simulink model "bary_source_seeking"  (R2017a)
settings: Solver=ode4  StartTime=0  StopTime=tf  FixedStep=1e-5  RelTol=1e-3
values from neighbouring files (symbols this model uses):
  lambda = t/T    [gentrajmodel_2Drobot.m]    (also in main.m = 1; sim_model.m = 1; source_estimation.m = sestimation_info.lambda)
  nu = 10    [main.m]    (also in sim_model.m; source_estimation.m = sestimation_info.nu)
  SAT_CONTROL = 10    [main.m]    (also in sim_model.m)
  T_cur = 1    [main.m]    (also in run_control_law.m = sestimation_info.T_cur; sim_model.m)
  T_traj = 1    [main.m]    (also in run_control_law.m = trajectory_info.T_traj; sim_model.m)
  traj_type = 1    [main.m]    (also in sim_model.m)
  x0 = [2; 2; 0; 1; 1; 1]    [main.m]    (also in sim_model.m)
undefined symbols (not defined in the file or in its folder): devval, is_sat, v_max, v_min, w_max
settings Model: Creator=brunolnetto  LastModifiedBy=brunolnetto

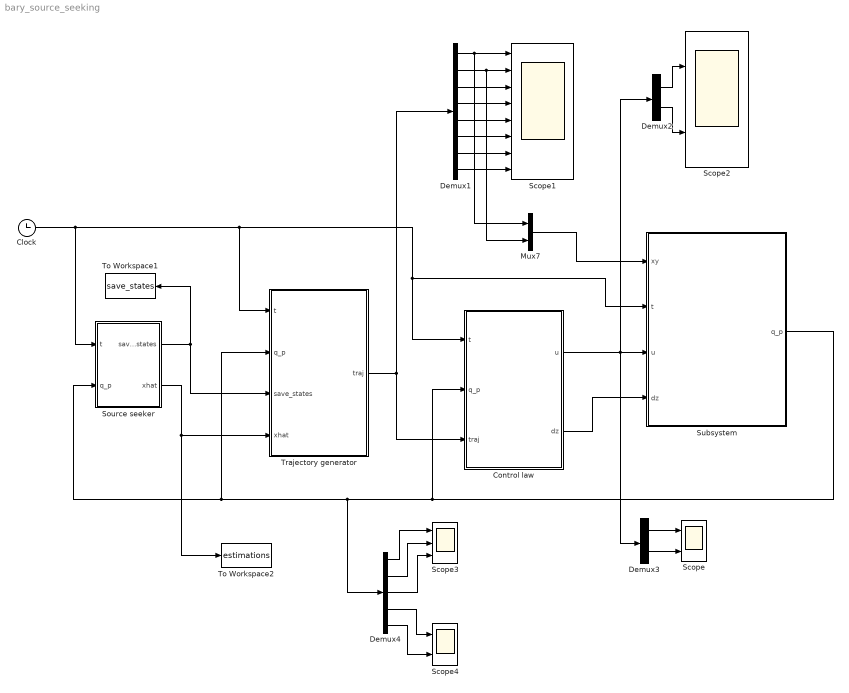
== system bary_source_seeking ==
  Clock : Clock
  Control law : MATLAB Function  TreatAsAtomicUnit=on
  Demux1 : Demux  Outputs=8
  Demux2 : Demux  Outputs=2
  Demux3 : Demux  Outputs=2
  Demux4 : Demux  Outputs=5
  Mux7 : Mux  Inputs=2
  Scope : Scope  NumInputPorts=2
  Scope1 : Scope  NumInputPorts=8
  Scope2 : Scope  NumInputPorts=2
  Scope3 : Scope  NumInputPorts=3
  Scope4 : Scope  NumInputPorts=2
  Source seeker : Subsystem
  Subsystem : Subsystem
  To Workspace1 : ToWorkspace  VariableName=save_states  SaveFormat=Structure With Time  SampleTime=-1
  To Workspace2 : ToWorkspace  VariableName=estimations  SaveFormat=Structure With Time  SampleTime=-1
  Trajectory generator : Subsystem
  wires:
  Clock/1 -> Control law/1(t), Subsystem/2(t), Trajectory generator/1(t), Source seeker/1(t)
  Demux1/3 -> Scope1/3
  Demux1/4 -> Scope1/4
  Demux1/5 -> Scope1/5
  Demux1/6 -> Scope1/6
  Demux1/7 -> Scope1/7
  Demux1/8 -> Scope1/8
  Demux1/2 -> Scope1/2, Mux7/2
  Demux1/1 -> Scope1/1, Mux7/1
  Mux7/1 -> Subsystem/1(xy)
  Control law/2(dz) -> Subsystem/4(dz)
  Source seeker/1(save_states) -> To Workspace1/1, Trajectory generator/3(save_states)
  Source seeker/2(xhat) -> Trajectory generator/4(xhat), To Workspace2/1
  Control law/1(u) -> Demux3/1, Demux2/1, Subsystem/3(u)
  Demux2/1 -> Scope2/1
  Demux2/2 -> Scope2/2
  Trajectory generator/1(traj) -> Demux1/1, Control law/3(traj)
  Demux3/1 -> Scope/1
  Demux3/2 -> Scope/2
  Subsystem/1(q_p) -> Control law/2(q_p), Demux4/1, Trajectory generator/2(q_p), Source seeker/2(q_p)
  Demux4/1 -> Scope3/1
  Demux4/2 -> Scope3/2
  Demux4/3 -> Scope3/3
  Demux4/4 -> Scope4/1
  Demux4/5 -> Scope4/2

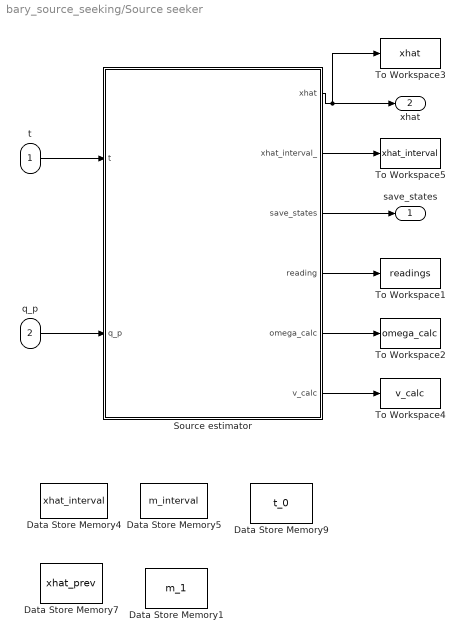
== system bary_source_seeking/Source seeker ==
  t : Inport
  q_p : Inport  Port=2
  Data Store Memory1 : DataStoreMemory  DataStoreName=m_1  ReadBeforeWriteMsg=warning  WriteAfterWriteMsg=warning  WriteAfterReadMsg=warning  ShowAdditionalParam=off  OutDataTypeStr=double
  Data Store Memory4 : DataStoreMemory  DataStoreName=xhat_interval  ReadBeforeWriteMsg=warning  WriteAfterWriteMsg=warning  WriteAfterReadMsg=warning  InitialValue=xhat0  ShowAdditionalParam=off  OutDataTypeStr=double  Dimensions=[2, 1]
  Data Store Memory5 : DataStoreMemory  DataStoreName=m_interval  ReadBeforeWriteMsg=warning  WriteAfterWriteMsg=warning  WriteAfterReadMsg=warning  ShowAdditionalParam=off  OutDataTypeStr=double
  Data Store Memory7 : DataStoreMemory  DataStoreName=xhat_prev  ReadBeforeWriteMsg=warning  WriteAfterWriteMsg=warning  WriteAfterReadMsg=warning  InitialValue=xhat0  ShowAdditionalParam=off  OutDataTypeStr=double
  Data Store Memory9 : DataStoreMemory  DataStoreName=t_0  ReadBeforeWriteMsg=warning  WriteAfterWriteMsg=warning  WriteAfterReadMsg=warning  ShowAdditionalParam=off  OutDataTypeStr=double
  Source estimator : MATLAB Function  TreatAsAtomicUnit=on
  To Workspace1 : ToWorkspace  VariableName=readings  SaveFormat=Structure With Time  SampleTime=-1
  To Workspace2 : ToWorkspace  VariableName=omega_calc  SaveFormat=Structure With Time  SampleTime=-1
  To Workspace3 : ToWorkspace  VariableName=xhat  SaveFormat=Structure With Time  SampleTime=-1
  To Workspace4 : ToWorkspace  VariableName=v_calc  SaveFormat=Structure With Time  SampleTime=-1
  To Workspace5 : ToWorkspace  VariableName=xhat_interval  SaveFormat=Structure With Time  SampleTime=-1
  save_states : Outport
  xhat : Outport  Port=2
  wires:
  Source estimator/4(reading) -> To Workspace1/1
  Source estimator/5(omega_calc) -> To Workspace2/1
  Source estimator/1(xhat) -> xhat/1, To Workspace3/1
  Source estimator/6(v_calc) -> To Workspace4/1
  t/1 -> Source estimator/1(t)
  q_p/1 -> Source estimator/2(q_p)
  Source estimator/3(save_states) -> save_states/1
  Source estimator/2(xhat_interval_) -> To Workspace5/1

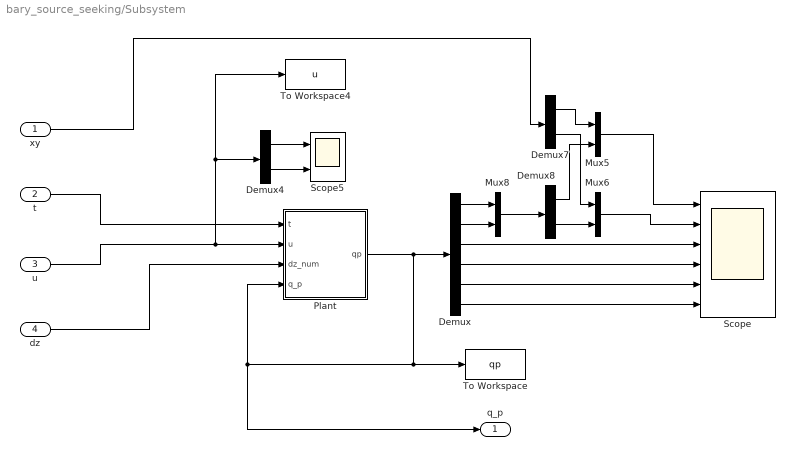
== system bary_source_seeking/Subsystem ==
  xy : Inport
  t : Inport  Port=2
  u : Inport  Port=3
  dz : Inport  Port=4
  Demux : Demux  Outputs=6
  Demux4 : Demux  Outputs=2
  Demux7 : Demux  Outputs=2
  Demux8 : Demux  Outputs=2
  Mux5 : Mux  Inputs=2
  Mux6 : Mux  Inputs=2
  Mux8 : Mux  Inputs=2
  Plant : Subsystem
  Scope : Scope  NumInputPorts=6
  Scope5 : Scope  NumInputPorts=2
  To Workspace : ToWorkspace  VariableName=qp  SaveFormat=Structure With Time  SampleTime=-1
  To Workspace4 : ToWorkspace  VariableName=u  SaveFormat=Structure With Time  SampleTime=-1
  q_p : Outport
  wires:
  t/1 -> Plant/1(t)
  Demux/3 -> Scope/3
  Demux/4 -> Scope/4
  Demux/5 -> Scope/5
  Demux/6 -> Scope/6
  Demux4/1 -> Scope5/1
  Demux4/2 -> Scope5/2
  Mux6/1 -> Scope/2
  Demux8/2 -> Mux6/2
  Demux7/2 -> Mux6/1
  Demux8/1 -> Mux5/2
  Demux7/1 -> Mux5/1
  Mux5/1 -> Scope/1
  xy/1 -> Demux7/1
  Demux/1 -> Mux8/1
  Demux/2 -> Mux8/2
  Mux8/1 -> Demux8/1
  Plant/1(qp) -> To Workspace/1, q_p/1, Plant/4(q_p), Demux/1
  dz/1 -> Plant/3(dz_num)
  u/1 -> Plant/2(u), To Workspace4/1, Demux4/1

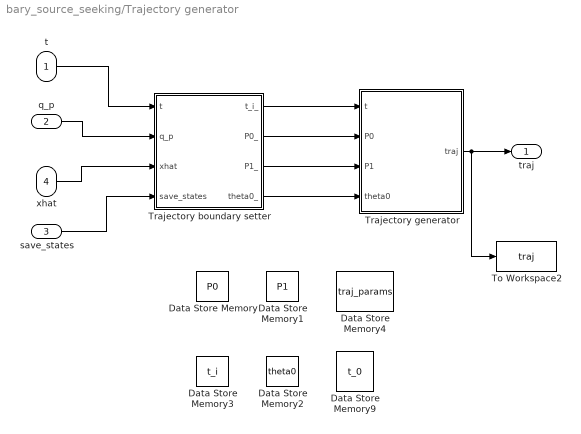
== system bary_source_seeking/Trajectory generator ==
  t : Inport
  q_p : Inport  Port=2
  save_states : Inport  Port=3
  xhat : Inport  Port=4
  Data Store Memory : DataStoreMemory  DataStoreName=P0  ReadBeforeWriteMsg=warning  WriteAfterWriteMsg=warning  WriteAfterReadMsg=warning  InitialValue=x0(1:2)  ShowAdditionalParam=off  OutDataTypeStr=double  Dimensions=[2, 1]
  Data Store Memory1 : DataStoreMemory  DataStoreName=P1  ReadBeforeWriteMsg=warning  WriteAfterWriteMsg=warning  WriteAfterReadMsg=warning  InitialValue=xhat0  ShowAdditionalParam=off  OutDataTypeStr=double
  Data Store Memory2 : DataStoreMemory  DataStoreName=theta0  ReadBeforeWriteMsg=warning  WriteAfterWriteMsg=warning  WriteAfterReadMsg=warning  InitialValue=x0(3)  ShowAdditionalParam=off  OutDataTypeStr=double
  Data Store Memory3 : DataStoreMemory  DataStoreName=t_i  ReadBeforeWriteMsg=warning  WriteAfterWriteMsg=warning  WriteAfterReadMsg=warning  ShowAdditionalParam=off  OutDataTypeStr=double
  Data Store Memory4 : DataStoreMemory  DataStoreName=traj_params  ReadBeforeWriteMsg=warning  WriteAfterWriteMsg=warning  WriteAfterReadMsg=warning  ShowAdditionalParam=off  OutDataTypeStr=double
  Data Store Memory9 : DataStoreMemory  DataStoreName=t_0  ReadBeforeWriteMsg=warning  WriteAfterWriteMsg=warning  WriteAfterReadMsg=warning  ShowAdditionalParam=off  OutDataTypeStr=double
  To Workspace2 : ToWorkspace  VariableName=traj  SaveFormat=Structure With Time  SampleTime=-1
  Trajectory boundary setter : MATLAB Function  TreatAsAtomicUnit=on
  Trajectory generator : MATLAB Function  TreatAsAtomicUnit=on
  traj : Outport
  wires:
  Trajectory boundary setter/4(theta0_) -> Trajectory generator/4(theta0)
  Trajectory boundary setter/2(P0_) -> Trajectory generator/2(P0)
  q_p/1 -> Trajectory boundary setter/2(q_p)
  Trajectory generator/1(traj) -> traj/1, To Workspace2/1
  t/1 -> Trajectory boundary setter/1(t)
  save_states/1 -> Trajectory boundary setter/4(save_states)
  Trajectory boundary setter/3(P1_) -> Trajectory generator/3(P1)
  Trajectory boundary setter/1(t_i_) -> Trajectory generator/1(t)
  xhat/1 -> Trajectory boundary setter/3(xhat)

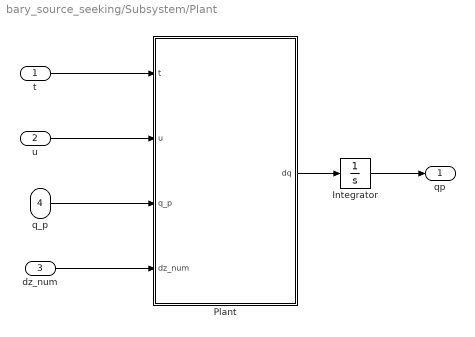
== system bary_source_seeking/Subsystem/Plant ==
  t : Inport
  u : Inport  Port=2
  dz_num : Inport  Port=3
  q_p : Inport  Port=4
  Integrator : Integrator  InitialCondition=x0
  Plant : MATLAB Function  TreatAsAtomicUnit=on
  qp : Outport
  wires:
  q_p/1 -> Plant/3(q_p)
  Plant/1(dq) -> Integrator/1
  Integrator/1 -> qp/1
  dz_num/1 -> Plant/4(dz_num)
  t/1 -> Plant/1(t)
  u/1 -> Plant/2(u)

== matlab function bary_source_seeking/Subsystem/Plant/Plant ==
  data: dq output; t input; u input; q_p input; dz_num input
function dq = plant(t, u, q_p, dz_num) 

	u_1 = u(1); 
	u_2 = u(2); 
	x_1 = q_p(1); 
	x_2 = q_p(2); 
	x_3 = q_p(3); 
	x_4 = q_p(4); 
	x_5 = q_p(5);dq = [x_4.*cos(x_3);x_4.*sin(x_3);x_5;u_1.*3.03030303030303e1+u_2.*3.03030303030303e1;u_1.*2.323447457256143e2-u_2.*2.323447457256143e2; dz_num];

== matlab function bary_source_seeking/Control law ==
  data: t input; u output; q_p input; traj input; dz output; T_cur parameter; T_traj parameter; SAT_CONTROL parameter; is_sat parameter
function [u, dz] = run_control_law(t, q_p, traj, T_cur, T_traj, SAT_CONTROL, is_sat)

	if(T_traj < T_cur)
			error('Trajectory plan time span must be greater than curiosity time');
	end

	x_1 = q_p(1);
	x_2 = q_p(2);
	x_3 = q_p(3);
	x_4 = q_p(4);
	x_5 = q_p(5);
	x_6 = q_p(6);
	x_pos_ref = traj(1);
	y_pos_ref = traj(2);
	xp_ref = traj(3);
	yp_ref = traj(4);
	xpp_ref = traj(5);
	ypp_ref = traj(6);
	xppp_ref = traj(7);
	yppp_ref = traj(8);

t2 = 1.0./x_4;
t3 = cos(x_3);
t4 = sin(x_3);
t5 = x_6.*1.65e-2;
u = [t5-x_5.*3.868043924382663e-2-t2.*t3.*x_2.*4.628455899988937e-1+t2.*t4.*x_1.*4.628455899988937e-1-t2.*t4.*x_pos_ref.*4.628455899988937e-1-t2.*t4.*xp_ref.*2.317524803959515e-1-t2.*t4.*xpp_ref.*3.868043924382663e-2-t2.*t4.*xppp_ref.*2.151974637681159e-3+t2.*t3.*y_pos_ref.*4.628455899988937e-1+t2.*t3.*yp_ref.*2.317524803959515e-1+t2.*t3.*ypp_ref.*3.868043924382663e-2+t2.*t3.*yppp_ref.*2.151974637681159e-3-t2.*x_5.*x_6.*4.303949275362318e-3;t5+x_5.*3.868043924382663e-2+t2.*t3.*x_2.*4.628455899988937e-1-t2.*t4.*x_1.*4.628455899988937e-1+t2.*t4.*x_pos_ref.*4.628455899988937e-1+t2.*t4.*xp_ref.*2.317524803959515e-1+t2.*t4.*xpp_ref.*3.868043924382663e-2+t2.*t4.*xppp_ref.*2.151974637681159e-3-t2.*t3.*y_pos_ref.*4.628455899988937e-1-t2.*t3.*yp_ref.*2.317524803959515e-1-t2.*t3.*ypp_ref.*3.868043924382663e-2-t2.*t3.*yppp_ref.*2.151974637681159e-3+t2.*x_5.*x_6.*4.303949275362318e-3];


	if(is_sat) 
		for i = 1:length(u)
			if(abs(u(i)) > SAT_CONTROL) 
				u(i) = sign(u(i))*SAT_CONTROL; 
			end 
		end 
	end

t2 = cos(x_3);
t3 = sin(x_3);
dz = x_4.*-1.076929422577556e2-x_6.*1.797439364132395e1-t2.*x_1.*2.150794818370298e2-t3.*x_2.*2.150794818370298e2+t2.*x_pos_ref.*2.150794818370298e2+t2.*xp_ref.*1.076929422577556e2+t2.*xpp_ref.*1.797439364132395e1+t2.*xppp_ref+t3.*y_pos_ref.*2.150794818370298e2+t3.*yp_ref.*1.076929422577556e2+t3.*ypp_ref.*1.797439364132395e1+t3.*yppp_ref+x_4.*x_5.^2;

== matlab function bary_source_seeking/Source seeker/Source estimator ==
  data: t input; xhat output; xhat_interval_ output; q_p input; save_states output; nu parameter; lambda parameter; T_cur parameter; v_min parameter; xhat_interval data_store_memory; m_interval data_store_memory; xhat_prev data_store_memory; t_0 data_store_memory; m_1 data_store_memory; v_max parameter; w_max parameter; devval parameter; reading output; omega_calc output; v_calc output
function [xhat, xhat_interval_, save_states, reading, omega_calc, v_calc] = ...
          source_estimation(t, q_p, nu, lambda, T_cur, ...
                            v_min, v_max, w_max, devval)
    
    global t_0 xhat_prev m_interval xhat_interval;
    persistent v_calc_curr omega_calc_curr;
    
    if(isempty(v_calc_curr))
        v_calc_curr = zeros(size(2, 1));
    end
    
    if(isempty(omega_calc_curr))
        omega_calc_curr = zeros(size(2, 1));
    end
    
    oracle = @(x) x(1)^2 + x(2)^2;
    
    x_curr = q_p(1:2, 1);
    theta_curr = q_p(3, 1);
    e_i = exp(-nu*oracle(x_curr));
    
    n = length(x_curr);
    
    % Update source estimation window
    delta_T = t - t_0;
    if(delta_T > T_cur)
        % Quick hack: Avoid multiple reads of runge-kutta algorithm
        t_0 = t;
        
        % TAKE NOTE: zero xs_curr to reduce number of operations and storage
        orient_curr = [cos(theta_curr); sin(theta_curr)];
        x_curr = q_p(1:2);
        
        [xhat, omega_calc, v_calc] = ...
            feasible_normrnd(x_curr, orient_curr, xhat_interval, ...
                             T_cur, v_min, v_max, w_max, devval);
        
        xhat_prev = xhat;
        
        v_calc_curr = v_calc;
        omega_calc_curr = omega_calc;
        
        save_states = true;
    else
        save_states = false;
    end
    
    xhat = xhat_prev;
    x_curr = q_p(1:2);
    
    xhat_interval = (lambda*m_interval*xhat_interval + x_curr*e_i)/(lambda*m_interval + e_i);
    m_interval = m_interval + e_i;
    
    omega_calc = omega_calc_curr;
    v_calc = v_calc_curr;
    reading = oracle(x_curr);
    xhat = xhat_interval;
    xhat_interval_ = xhat_interval;
end

== matlab function bary_source_seeking/Trajectory generator/Trajectory boundary setter ==
  data: t_i_ output; P0_ output; P1_ output; theta0_ output; t input; q_p input; xhat input; save_states input; t_0 data_store_memory; P0 data_store_memory; P1 data_store_memory; theta0 data_store_memory
function [t_i_, P0_, P1_, theta0_] = trajectory(t, q_p, xhat, save_states)
    global P0 P1 t_0 theta0;
    
    if(save_states)
        t_0 = t;
        
        P0 = q_p(1:2);
        P1 = xhat;
        
        theta0 = q_p(3);
        
        t_i = t - t_0;
    end
    
    P0_ = P0;
    P1_ = P1;
    theta0_ = theta0;
    t_i_ = t - t_0;
end

== matlab function bary_source_seeking/Trajectory generator/Trajectory generator ==
  data: t input; P0 input; P1 input; theta0 input; T_traj parameter; traj output size=[8, 1]; traj_params data_store_memory; traj_type parameter
function traj = traj_gen(t, P0, P1, theta0, T_traj, traj_type)
    P0 = double(P0);
    P1 = double(P1);
    
    T = T_traj;
    
    switch traj_type
        case 1
            xy_t = P0 + (t/T)*(P1 - P0);
            dxy_t = (P1 - P0)/T;
            d2xy_t = zeros(size(P0));
            d3xy_t = zeros(size(P0));            
            
            traj = [xy_t; dxy_t; d2xy_t; d3xy_t];
            
        case 2    
            % TAKE NOTE: MUST be lesser than 1
            % one may adjust
            alpha0 = 0.3;
            alpha1 = 0.3;

            P0_prev = P0;

            % Exponential and polynomial curves
            xy_t = bezier_path(t, T, P0, P1, theta0, alpha0, alpha1);
            dxy_t = dbezier_path(t, T, P0, P1, theta0, alpha0, alpha1, 1);
            d2xy_t = dbezier_path(t, T, P0, P1, theta0, alpha0, alpha1, 2);
            d3xy_t = dbezier_path(t, T, P0, P1, theta0, alpha0, alpha1, 3);
            
            traj = [xy_t; dxy_t; d2xy_t; d3xy_t];
            
%         case 3
%             v = norm(P1 - P0)/T;
%             
%             % Percentage under AB distance
%             alpha_0 = 0.2;
%             alpha_1 = 0.2;
%             
%             [~, dAB, ~, ~, ~] = ...
%              traj_tangentAB_sim(t, P0, P1, theta0, ...
%                                 v, alpha_0, alpha_1);
%             
%             % Circle radius
%             v = dAB/T_cur;
%             
%             [traj, ~, ~, ~, ~] = ...
%             traj_tangentAB_sim(t, P0, P1, theta0, v, alpha_0, alpha_1);
    
        otherwise
            error('Must be either 1 or 2.')
    end
    
end

% function traj = traj_gen(t, P0, P1, theta0, T_cur, traj_type)
%     P0 = double(P0);
%     P1 = double(P1);
%     
%     T = T_cur;
%     
%     traj = [];
%     
%     switch traj_type
%         case 1
%             xy_t = P0 + (t/T)*(P1 - P0);
%             dxy_t = (P1 - P0)/T;
%             d2xy_t = zeros(size(P0));
%             d3xy_t = zeros(size(P0));            
%             
%             traj = [xy_t; dxy_t; d2xy_t; d3xy_t];
%             
%         case 2    
%             % TAKE NOTE: MUST be lesser than 1
%             % one may adjust
%             alpha0 = 0.3;
%             alpha1 = 0.3;
% 
%             P0_prev = P0;
% 
%             % Exponential and polynomial curves
%             xy_t = bezier_path(t, T, P0, P1, theta0, alpha0, alpha1);
%             dxy_t = dbezier_path(t, T, P0, P1, theta0, alpha0, alpha1, 1);
%             d2xy_t = dbezier_path(t, T, P0, P1, theta0, alpha0, alpha1, 2);
%             d3xy_t = dbezier_path(t, T, P0, P1, theta0, alpha0, alpha1, 3);
%             
%             traj = [xy_t; dxy_t; d2xy_t; d3xy_t];
%             
%         case 3
%             v = norm(P1 - P0)/T;
% 
%             v_0 = v;
%             v_01 = v; 
%             v_1 = v;
% 
%             % Percentage under AB distance
%             alpha_0 = 0.2;
%             alpha_1 = 0.2;
%                         
%             [~, dAB, ~, ~, ~] = ...
%              traj_tangentAB_sim(P0, P1, theta0, ...
%                                 v_0, v_01, v_1, ...
%                                 alpha_0, alpha_1);
%             
%             % Distance between path points
%             BA = P1 - P0;
% 
%             % Circle radius
%             v = dAB/T_cur;
%             v_0 = v;
%             v_01 = v;
%             v_1 = v;
% 
%             [traj, ~, ~, ~, ~] = ...
%             traj_tangentAB_sim(P0, P1, theta0, ...
%                                v_0, v_01, v_1, ...
%                                alpha_0, alpha_1);
%     
%         otherwise
%             error('Must be either 1 or 2.')
%     end
%     
% %     switch traj_type
% %         case 1
% %             xy_t = P0 + (t/T)*(P1 - P0);
% %             dxy_t = (P1 - P0)/T;
% %             d2xy_t = zeros(size(P0));
% %             d3xy_t = zeros(size(P0));
% %             
% %         case 2
% %             % TAKE NOTE: MUST be lesser than 1
% %             % one may adjust
% %             alpha0 = 0.3;
% %             alpha1 = 0.3;
% % 
% %             P0_prev = P0;
% % 
% %             % Exponential and polynomial curves
% %             xy_t = bezier_path(t, T, P0, P1, theta0, alpha0, alpha1);
% %             dxy_t = dbezier_path(t, T, P0, P1, theta0, alpha0, alpha1, 1);
% %             d2xy_t = dbezier_path(t, T, P0, P1, theta0, alpha0, alpha1, 2);
% %             d3xy_t = dbezier_path(t, T, P0, P1, theta0, alpha0, alpha1, 3);
% %             
% %         case 3
% %             P0_prev = P0;
% %             
% %             alpha = 0.5;
% %             traj_params.xy_t = traj_exppoly(t, P0, P1, theta0, alpha, T, 'poly');
% % 
% %             dxy_t = diff(traj_params.xy_t, t_);
% %             d2xy_t = diff(dxy_t, t_);
% %             d3xy_t = diff(d2xy_t, t_);
% %             
% %         case 4
% %             P0_prev = P0;
% %             
% %             alpha = 0.5;
% %             traj_params.xy_t = traj_exppoly(t, P0, P1, theta0, alpha, T, 'exp');
% %             
% %             dxy_t = diff(traj_params.xy_t, t_);
% %             d2xy_t = diff(dxy_t, t_);
% %             d3xy_t = diff(d2xy_t, t_);
% %             
% %         case 5
% %             P0_prev = P0;
% %             traj_params = struct('');
% % 
% %             v = norm(P1 - P0)/T;
% % 
% %             v_0 = v;
% %             v_01 = v; 
% %             v_1 = v;
% % 
% %             % Percentage under AB distance
% %             alpha_0 = 0.2;
% %             alpha_1 = 0.2;
% % 
% %             traj_params = traj_tangentAB(P0, P1, theta0, ...
% %                                          v_0, v_01, v_1, ...
% %                                          alpha_0, alpha_1);
% % 
% %             % Geometrical properties
% %             arg0 = traj_params.arg0;
% %             dCD = traj_params.dCD;
% %             arg1 = traj_params.arg1;
% % 
% %             r0 = traj_params.r0;
% %             r1 = traj_params.r1;
% % 
% %             v = (r0*arg0 + dCD + r1*arg1)/T;
% %             v_0 = v;
% %             v_01 = v;
% %             v_1 = v;
% % 
% %             t_0 = traj_params.t_0;
% %             t_01 = traj_params.t_01;
% %             t_1 = traj_params.t_1;
% % 
% %             traj_params = traj_tangentAB(P0, P1, theta0, v_0, v_01, v_1, alpha_0, alpha_1);
% %             
% %             dxy_t = diff(traj_params.xy_t, t_);
% %             d2xy_t = diff(dxy_t, t_);
% %             d3xy_t = diff(d2xy_t, t_);
% %     end
% 
% end
